simulink model "Sample594"  (R2021b)
settings: Solver=VariableStepAuto  StartTime=0.0  StopTime=10.0  RelTol=1e-3
undefined symbols (not defined in the file): DiscIntNeverNeededParam, magnitude, Newton, Raphson
libraries: simulink x402, pid_lib x98
(part 4 of 14)

== system Sample594/cfblk7/cfblk12/cfblk8 ==
  cfblk1 : Inport
  cfblk8 : Inport  Port=2
  cfblk10 : Subsystem  TreatAsAtomicUnit=on
  cfblk{11..14} (4 alike) : Delay  SampleTime=1
  cfblk3 : simulink/Discrete/Transfer Fcn Lead or Lag  PoleZ=0.95  ZeroZ=0.75  ICPrevOutput=0.0  ICPrevInput=0.0  DoSatur=off
      settings: SourceProductBaseCode=SL
  cfblk4 : DiscreteFir  SampleTime=1
  cfblk5 : Bias  Bias=[232401937.403829]
  cfblk6 : Subsystem
  cfblk7 : If  IfExpression=u1 >= 0  SampleTime=1
  cfblk9 : Subsystem  TreatAsAtomicUnit=on
  cfblk2 : Outport
  wires:
  cfblk1/1 -> cfblk5/1
  cfblk8/1 -> cfblk3/1
  cfblk5/1 -> cfblk4/1, cfblk9/3(cfblk7)
  cfblk3/1 -> cfblk2/1
  cfblk9/1(cfblk2) -> cfblk6/1(cfblk1)
  cfblk4/1 -> cfblk9/2(cfblk6)
  cfblk6/1(cfblk2) -> cfblk11/1, cfblk14/1
  cfblk7/1 -> cfblk9/Action
  cfblk7/2 -> cfblk10/Action
  cfblk11/1 -> cfblk10/1(cfblk1)
  cfblk10/1(cfblk2) -> cfblk12/1
  cfblk12/1 -> cfblk9/1(cfblk1)
  cfblk10/2(cfblk10) -> cfblk13/1
  cfblk13/1 -> cfblk7/1
  cfblk14/1 -> cfblk9/4(cfblk8)

== system Sample594/cfblk7/cfblk12/cfblk9 ==
  cfblk1 : Inport
  cfblk10 : Inport  Port=2
  cfblk11 : Delay  SampleTime=1
  cfblk12 : Delay  SampleTime=1
  cfblk3 : simulink/Discrete/Transfer Fcn First Order  PoleZ=0.95  ICPrevOutput=0.0  DoSatur=off
  cfblk4 : simulink/Discrete/Transfer Fcn First Order  PoleZ=0.95  ICPrevOutput=0.0  DoSatur=off
  cfblk5 : Gain  Gain=[219422416.424969]
  cfblk6 : Polyval  Coefs=[ +2.081618890e-019, -1.441693666e-014, +4.719686976e-010, -8.536869453e-006, +1.621573104e-001, -8.087801117e+001 ]
  cfblk7 : Rounding
  cfblk8 : Constant  Value=[284617864.400396]  SampleTime=1
  cfblk9 : Subsystem
  cfblk2 : Outport
  wires:
  cfblk3/1 -> cfblk5/1
  cfblk1/1 -> cfblk3/1
  cfblk9/1(cfblk2) -> cfblk7/1
  cfblk4/1 -> cfblk9/1(cfblk1)
  cfblk7/1 -> cfblk6/1
  cfblk8/1 -> cfblk2/1
  cfblk6/1 -> cfblk11/1
  cfblk11/1 -> cfblk9/2(cfblk12)
  cfblk9/2(cfblk13) -> cfblk12/1
  cfblk12/1 -> cfblk4/1

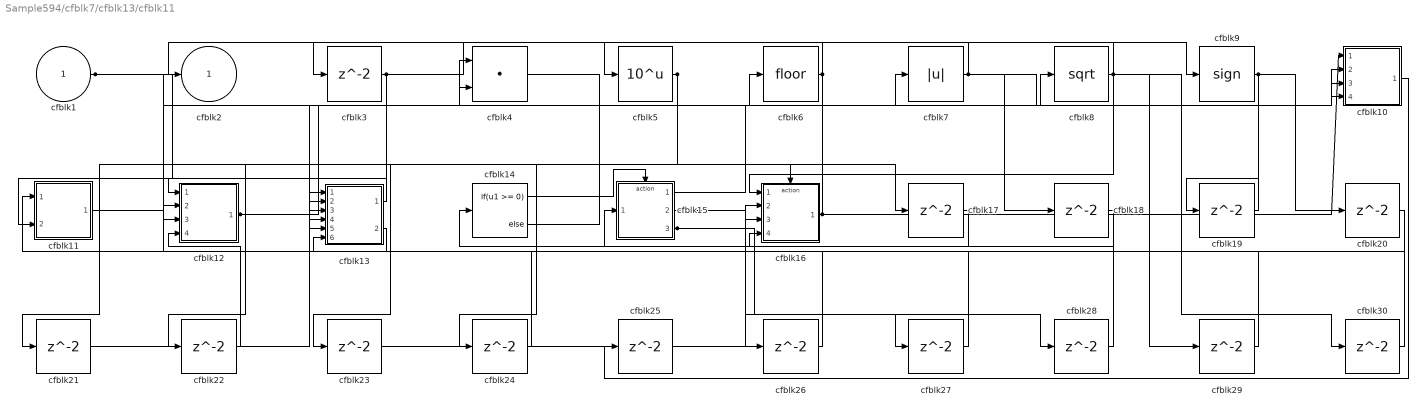
== system Sample594/cfblk7/cfblk13/cfblk11 ==
  cfblk1 : Inport
  cfblk10 : Subsystem
  cfblk11 : Subsystem
  cfblk12 : Subsystem
  cfblk13 : Subsystem
  cfblk14 : If  IfExpression=u1 >= 0  SampleTime=1
  cfblk15 : Subsystem  TreatAsAtomicUnit=on
  cfblk16 : Subsystem  TreatAsAtomicUnit=on
  cfblk{3,17..30} (15 alike) : Delay  SampleTime=1
  cfblk4 : DotProduct  InputSameDT=on  OutDataTypeStr=Inherit: Inherit via internal rule
  cfblk5 : Math  Operator=10^u  SaturateOnIntegerOverflow=on
  cfblk6 : Rounding
  cfblk7 : Abs
  cfblk8 : Sqrt  SaturateOnIntegerOverflow=on
  cfblk9 : Signum
  cfblk2 : Outport
  wires:
  cfblk12/1(cfblk2) -> cfblk8/1, cfblk10/2(cfblk13)
  cfblk8/1 -> cfblk16/1(cfblk1), cfblk2/1, cfblk29/1, cfblk30/1
  cfblk3/1 -> cfblk9/1, cfblk11/2(cfblk7)
  cfblk15/1(cfblk2) -> cfblk7/1
  cfblk16/1(cfblk2) -> cfblk4/1, cfblk10/1(cfblk1)
  cfblk13/1(cfblk2) -> cfblk12/1(cfblk1)
  cfblk13/2(cfblk17) -> cfblk11/1(cfblk1)
  cfblk11/1(cfblk2) -> cfblk6/1
  cfblk6/1 -> cfblk5/1, cfblk21/1, cfblk22/1
  cfblk15/3(cfblk7) -> cfblk27/1, cfblk28/1
  cfblk7/1 -> cfblk3/1, cfblk10/3(cfblk14), cfblk18/1
  cfblk5/1 -> cfblk23/1, cfblk24/1
  cfblk1/1 -> cfblk13/3(cfblk13), cfblk10/4(cfblk15)
  cfblk9/1 -> cfblk19/1, cfblk20/1
  cfblk14/1 -> cfblk15/Action
  cfblk14/2 -> cfblk16/Action
  cfblk4/1 -> cfblk17/1
  cfblk17/1 -> cfblk15/1(cfblk1)
  cfblk18/1 -> cfblk14/1
  cfblk19/1 -> cfblk4/2
  cfblk20/1 -> cfblk13/6(cfblk16)
  cfblk21/1 -> cfblk13/2(cfblk12)
  cfblk22/1 -> cfblk12/4(cfblk14)
  cfblk23/1 -> cfblk16/3(cfblk11)
  cfblk24/1 -> cfblk13/5(cfblk15)
  cfblk10/1(cfblk2) -> cfblk25/1
  cfblk25/1 -> cfblk16/2(cfblk10)
  cfblk15/2(cfblk6) -> cfblk26/1
  cfblk26/1 -> cfblk13/1(cfblk1)
  cfblk27/1 -> cfblk12/2(cfblk12)
  cfblk28/1 -> cfblk16/4(cfblk12)
  cfblk29/1 -> cfblk12/3(cfblk13)
  cfblk30/1 -> cfblk13/4(cfblk14)

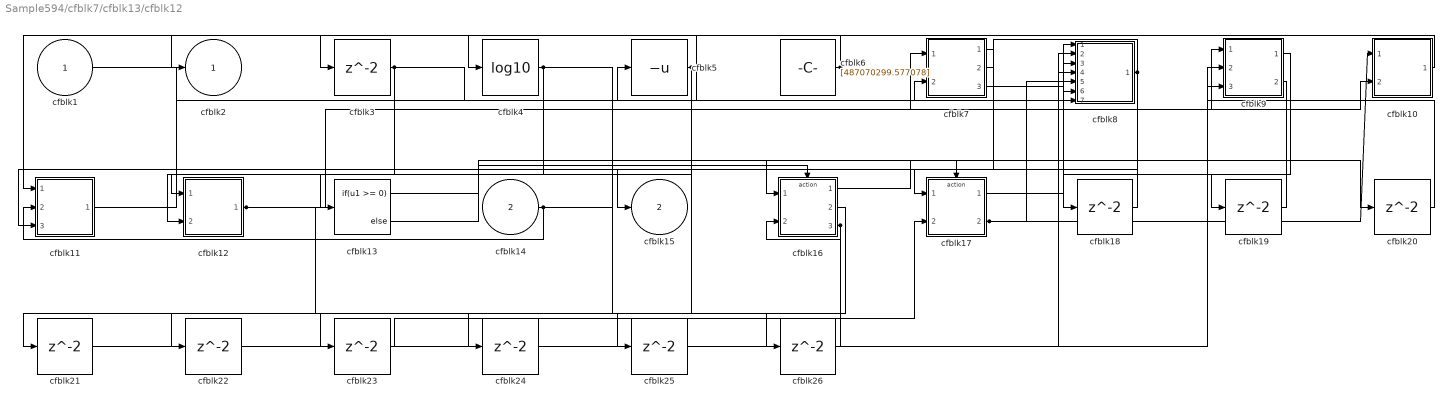
== system Sample594/cfblk7/cfblk13/cfblk12 ==
  cfblk1 : Inport
  cfblk14 : Inport  Port=2
  cfblk10 : Subsystem
  cfblk11 : Subsystem
  cfblk12 : Subsystem
  cfblk13 : If  IfExpression=u1 >= 0  SampleTime=1
  cfblk16 : Subsystem  TreatAsAtomicUnit=on
  cfblk17 : Subsystem  TreatAsAtomicUnit=on
  cfblk{3,18..26} (10 alike) : Delay  SampleTime=1
  cfblk4 : Math  Operator=log10  SaturateOnIntegerOverflow=on
  cfblk5 : UnaryMinus
  cfblk6 : Constant  Value=[487070299.577078]  SampleTime=1
  cfblk7 : Subsystem
  cfblk8 : Subsystem
  cfblk9 : Subsystem
  cfblk2 : Outport
  cfblk15 : Outport  Port=2
  wires:
  cfblk11/1(cfblk2) -> cfblk5/1
  cfblk12/1(cfblk2) -> cfblk9/1(cfblk1), cfblk24/1
  cfblk8/1(cfblk2) -> cfblk11/1(cfblk1), cfblk11/3(cfblk11)
  cfblk17/1(cfblk2) -> cfblk8/1(cfblk1)
  cfblk3/1 -> cfblk13/1, cfblk8/6(cfblk14)
  cfblk1/1 -> cfblk7/2(cfblk9)
  cfblk10/1(cfblk2) -> cfblk4/1
  cfblk6/1 -> cfblk2/1, cfblk3/1
  cfblk16/3(cfblk16) -> cfblk22/1, cfblk23/1
  cfblk4/1 -> cfblk12/1(cfblk1), cfblk26/1
  cfblk5/1 -> cfblk12/2(cfblk7), cfblk25/1
  cfblk7/1(cfblk2) -> cfblk17/1(cfblk1)
  cfblk17/2(cfblk9) -> cfblk10/1(cfblk1), cfblk8/5(cfblk13)
  cfblk14/1 -> cfblk11/2(cfblk10), cfblk10/2(cfblk8)
  cfblk7/2(cfblk10) -> cfblk15/1
  cfblk7/3(cfblk11) -> cfblk8/3(cfblk11)
  cfblk13/1 -> cfblk16/Action
  cfblk13/2 -> cfblk17/Action
  cfblk9/1(cfblk2) -> cfblk18/1
  cfblk18/1 -> cfblk7/1(cfblk1)
  cfblk9/2(cfblk8) -> cfblk19/1
  cfblk19/1 -> cfblk16/1(cfblk1)
  cfblk16/1(cfblk2) -> cfblk20/1
  cfblk20/1 -> cfblk9/2(cfblk6)
  cfblk16/2(cfblk15) -> cfblk21/1
  cfblk21/1 -> cfblk9/3(cfblk7)
  cfblk22/1 -> cfblk8/2(cfblk10)
  cfblk23/1 -> cfblk17/2(cfblk8)
  cfblk24/1 -> cfblk8/7(cfblk15)
  cfblk25/1 -> cfblk8/4(cfblk12)
  cfblk26/1 -> cfblk16/2(cfblk14)

== system Sample594/cfblk7/cfblk13/cfblk17 ==
  cfblk1 : Inport
  Action Port : ActionPort  ActionPortLabel=if(u1 >= 0)
  cfblk10 : Subsystem
  cfblk11 : Subsystem
  cfblk12 : Subsystem
  cfblk13 : Subsystem
  cfblk15 : Delay
  cfblk16 : Delay
  cfblk17 : Delay
  cfblk3 : simulink/Discrete/Difference  ICPrevInput=0.0  OutMin=[]  OutMax=[]  OutDataTypeStr=Inherit: Inherit via back propagation  OutDataType=fixdt(1, 16)  OutScaling=2^-10  DoSatur=off
  cfblk4 : DiscreteTransferFcn
  cfblk5 : Reshape
  cfblk6 : simulink/Math Operations/Slider Gain  gain=1  low=0  high=2
  cfblk7 : DotProduct  InputSameDT=on  OutDataTypeStr=Inherit: Inherit via internal rule
  cfblk8 : Constant  Value=[310623050.660394]  SampleTime=1
  cfblk9 : Subsystem
  cfblk2 : Outport
  cfblk14 : Outport  Port=2
  wires:
  cfblk6/1 -> cfblk11/1(cfblk1)
  cfblk13/1(cfblk2) -> cfblk3/1
  cfblk7/1 -> cfblk15/1, cfblk16/1
  cfblk3/1 -> cfblk2/1, cfblk7/2
  cfblk12/1(cfblk2) -> cfblk4/1, cfblk13/3(cfblk7)
  cfblk10/1(cfblk2) -> cfblk11/2(cfblk12)
  cfblk1/1 -> cfblk5/1, cfblk6/1, cfblk12/3(cfblk16)
  cfblk4/1 -> cfblk13/1(cfblk1), cfblk9/1(cfblk1)
  cfblk9/1(cfblk2) -> cfblk14/1
  cfblk11/1(cfblk2) -> cfblk12/1(cfblk1)
  cfblk5/1 -> cfblk10/2(cfblk7)
  cfblk8/1 -> cfblk13/2(cfblk6)
  cfblk9/3(cfblk10) -> cfblk7/1
  cfblk15/1 -> cfblk10/1(cfblk1)
  cfblk16/1 -> cfblk12/2(cfblk15)
  cfblk9/2(cfblk9) -> cfblk17/1
  cfblk17/1 -> cfblk11/3(cfblk13)

== system Sample594/cfblk7/cfblk13/cfblk18 ==
  cfblk1 : Inport
  Action Port : ActionPort  ActionPortLabel=else
  cfblk{9..12} (4 alike) : Delay
  cfblk3 : pid_lib/PID Controller  Controller=PID  Form=Parallel  TimeDomain=Discrete-time  UseExternalTs=off  SampleTime=-1  IntegratorMethod=Forward Euler  FilterMethod=Forward Euler  ControllerParametersSource=internal  P=1  I=1  D=0  UseFilter=on  N=100  TunerSelectOption=Transfer Function Based (PID Tuner App)  InitialConditionSource=internal  InitialConditionForIntegrator=0  InitialConditionForFilter=0  DifferentiatorICPrevScaledInput=0  ExternalReset=none  TrackingMode=off  Kt=1  LimitOutput=off  SatLimitsSource=internal  UpperSaturationLimit=inf  LowerSaturationLimit=-inf  LinearizeAsGain=off  AntiWindupMode=none  Kb=1  POutMin=[]  POutMax=[]  IOutMin=[]  IOutMax=[]  DOutMin=[]  DOutMax=[]  NOutMin=[]  NOutMax=[]  SumOutMin=[]  SumOutMax=[]  SaturationOutMin=[]  SaturationOutMax=[]  PParamMin=[]  PParamMax=[]  IParamMin=[]  IParamMax=[]  DParamMin=[]  DParamMax=[]  NParamMin=[]  NParamMax=[]  KbParamMin=[]  KbParamMax=[]  KtParamMin=[]  KtParamMax=[]  KbOutMin=[]  KbOutMax=[]  KtOutMin=[]  KtOutMax=[]  IntegratorOutMin=[]  IntegratorOutMax=[]  FilterOutMin=[]  FilterOutMax=[]  SumI1OutMin=[]  SumI1OutMax=[]  SumI2OutMin=[]  SumI2OutMax=[]  SumI3OutMin=[]  SumI3OutMax=[]  SumI4OutMin=[]  SumI4OutMax=[]  SumDOutMin=[]  SumDOutMax=[]  DifferentiatorOutMin=[]  DifferentiatorOutMax=[]  FilterDiffOutCoefMin=[]  FilterDiffOutCoefMax=[]  ReciprocalOutMin=[]  ReciprocalOutMax=[]  SumDenOutMin=[]  SumDenOutMax=[]  SumNumOutMin=[]  SumNumOutMax=[]  DivideOutMin=[]  DivideOutMax=[]  UdiffTsProdOutMin=[]  UdiffTsProdOutMax=[]  NTsProdOutMin=[]  NTsProdOutMax=[]  UintegralTsProdOutMin=[]  UintegralTsProdOutMax=[]  UngainTsProdOutMin=[]  UngainTsProdOutMax=[]  IntegratorContinuousStateAttributes=''  IntegratorStateMustResolveToSignalObject=off  IntegratorRTWStateStorageClass=Auto  FilterContinuousStateAttributes=''  FilterStateMustResolveToSignalObject=off  FilterRTWStateStorageClass=Auto  ParallelPVariant=InternalParameters  IdealPVariant=Disabled  IVariant=InternalParameters  DVariant=InternalParameters  IntegratorVariant=Discrete  SatVariant=Disabled  AWVariant=Passthrough  PCopyVariant=Disabled  TRVariant=Disabled  FdbkBlocksVariant=Forward  IdealPFdbkVariant=Disabled  SatFdbkVariant=Disabled  DerivativeFilterVariant=ForwardEulerFilter  NVariant=InternalParameters  NCopyVariant=Disabled  FilterICVariant=InternalICsFilter  IntegratorICVariant=InternalICs  ExternalResetVariant=Disabled  TRSumVariant=Passthrough  SumFdbkVariant=Disabled  SumVariant=Sum_PID  TsampFilterVariant=InternalTs  TsampNgainVariant=Passthrough  TsampIntegralVariant=Passthrough  ExternalSaturationOutDataTypeStr=Inherit: Same as second input
  cfblk4 : Assignment  DiagnosticForDimensions=Warning  IndexOptions=Index vector (dialog)  Indices=1  OutputSizes=1
  cfblk5 : Subsystem
  cfblk6 : Subsystem
  cfblk7 : Subsystem
  cfblk8 : Subsystem
  cfblk2 : Outport
  wires:
  cfblk1/1 -> cfblk5/1(cfblk1)
  cfblk7/1(cfblk2) -> cfblk4/2, cfblk9/1
  cfblk8/1(cfblk2) -> cfblk7/1(cfblk1), cfblk6/3(cfblk6)
  cfblk5/1(cfblk2) -> cfblk8/2(cfblk9)
  cfblk5/2(cfblk11) -> cfblk6/1(cfblk1), cfblk6/2(cfblk5), cfblk7/2(cfblk7), cfblk7/3(cfblk8), cfblk7/4(cfblk9)
  cfblk6/2(cfblk7) -> cfblk2/1, cfblk3/1, cfblk4/1
  cfblk9/1 -> cfblk5/3(cfblk9)
  cfblk4/1 -> cfblk10/1
  cfblk10/1 -> cfblk5/2(cfblk8)
  cfblk6/1(cfblk2) -> cfblk11/1
  cfblk11/1 -> cfblk8/1(cfblk1)
  cfblk3/1 -> cfblk12/1
  cfblk12/1 -> cfblk5/4(cfblk10)

== system Sample594/cfblk7/cfblk17/cfblk8 ==
  cfblk1 : Inport
  cfblk10 : MinMax  Function=max  Inputs=3
  cfblk11 : Gain  Gain=[-356507921.559494]
  cfblk12 : Constant  Value=[-799910356.310316]  SampleTime=1
  cfblk13 : Subsystem
  cfblk14 : Subsystem
  cfblk{15..18} (4 alike) : Delay
  cfblk3 : UnitDelay  SampleTime=-1  HasFrameUpgradeWarning=on
  cfblk4 : DiscreteStateSpace  SampleTime=-1
  cfblk5 : UnitDelay  SampleTime=-1  HasFrameUpgradeWarning=on
  cfblk6 : DiscreteStateSpace  SampleTime=-1
  cfblk7 : simulink/Discrete/Difference  ICPrevInput=0.0  OutMin=[]  OutMax=[]  OutDataTypeStr=Inherit: Inherit via back propagation  OutDataType=fixdt(1, 16)  OutScaling=2^-10  DoSatur=off
  cfblk8 : Gain  Gain=[-919229611.126287]
  cfblk9 : ComplexToMagnitudeAngle
  cfblk2 : Outport
  wires:
  cfblk5/1 -> cfblk6/1
  cfblk12/1 -> cfblk10/1
  cfblk4/1 -> cfblk7/1, cfblk11/1
  cfblk9/1 -> cfblk4/1
  cfblk3/1 -> cfblk14/1(cfblk1), cfblk13/3(cfblk14)
  cfblk11/1 -> cfblk10/2
  cfblk7/1 -> cfblk5/1
  cfblk8/1 -> cfblk13/2(cfblk13), cfblk18/1
  cfblk13/1(cfblk2) -> cfblk10/3
  cfblk9/2 -> cfblk8/1
  cfblk14/1(cfblk2) -> cfblk9/1
  cfblk6/1 -> cfblk13/1(cfblk1)
  cfblk1/1 -> cfblk2/1
  cfblk10/1 -> cfblk15/1
  cfblk15/1 -> cfblk3/1
  cfblk13/2(cfblk15) -> cfblk16/1
  cfblk16/1 -> cfblk14/3(cfblk10)
  cfblk13/3(cfblk16) -> cfblk17/1
  cfblk17/1 -> cfblk14/4(cfblk11)
  cfblk18/1 -> cfblk14/2(cfblk9)

== system Sample594/cfblk7/cfblk18/cfblk10 ==
  cfblk1 : Inport
  cfblk14 : Inport  Port=2
  cfblk15 : Inport  Port=3
  cfblk10 : Product
  cfblk11 : ComplexToMagnitudeAngle
  cfblk12 : Sqrt  Operator=rSqrt  AlgorithmType=Newton-Raphson  SaturateOnIntegerOverflow=on
  cfblk13 : Subsystem
  cfblk16 : Delay
  cfblk17 : Delay
  cfblk18 : Delay
  cfblk3 : Delay  ShowEnablePort=on
      settings: InputPortMap=u0,e6
  cfblk4 : simulink/Discrete/Transfer Fcn First Order  PoleZ=0.95  ICPrevOutput=0.0  DoSatur=off
  cfblk5 : DiscreteStateSpace  SampleTime=-1
  cfblk6 : DiscreteZeroPole  Poles=[0 0.5]  Gain=1  SampleTime=-1
  cfblk7 : DiscreteTransferFcn
  cfblk8 : Assignment  DiagnosticForDimensions=Warning  IndexOptions=Index vector (dialog)  Indices=1  OutputSizes=1
  cfblk9 : Sum  Inputs=+
  cfblk2 : Outport
  wires:
  cfblk13/1(cfblk2) -> cfblk5/1
  cfblk7/1 -> cfblk8/1
  cfblk6/1 -> cfblk9/1
  cfblk3/1 -> cfblk11/1
  cfblk10/1 -> cfblk6/1
  cfblk9/1 -> cfblk12/1
  cfblk5/1 -> cfblk7/1
  cfblk12/1 -> cfblk13/1(cfblk1)
  cfblk11/2 -> cfblk4/1
  cfblk8/1 -> cfblk3/2, cfblk17/1
  cfblk15/1 -> cfblk13/2(cfblk6)
  cfblk14/1 -> cfblk8/2
  cfblk4/1 -> cfblk2/1
  cfblk1/1 -> cfblk10/1
  cfblk11/1 -> cfblk16/1
  cfblk16/1 -> cfblk3/1
  cfblk17/1 -> cfblk13/3(cfblk7)
  cfblk13/2(cfblk8) -> cfblk18/1
  cfblk18/1 -> cfblk10/2

== system Sample594/cfblk7/cfblk18/cfblk9 ==
  cfblk1 : Inport
  cfblk10 : Subsystem
  cfblk3 : Delay  ShowEnablePort=on
      settings: InputPortMap=u0,e6
  cfblk4 : ComplexToRealImag
  cfblk5 : Abs
  cfblk6 : ComplexToMagnitudeAngle
  cfblk7 : Constant  Value=[389657295.438685]  SampleTime=1
  cfblk8 : Constant  Value=[-589872672.868971]  SampleTime=1
  cfblk9 : Constant  Value=[-970659271.621519]  SampleTime=1
  cfblk2 : Outport
  wires:
  cfblk4/1 -> cfblk3/1
  cfblk7/1 -> cfblk2/1
  cfblk8/1 -> cfblk5/1
  cfblk9/1 -> cfblk3/2
  cfblk5/1 -> cfblk10/1(cfblk1)
  cfblk1/1 -> cfblk6/1
  cfblk10/1(cfblk2) -> cfblk4/1

== system Sample594/cfblk7/cfblk19/cfblk7 ==
  cfblk1 : Inport
  cfblk11 : Inport  Port=2
  cfblk12 : Inport  Port=3
  cfblk10 : Constant  Value=[-662759039.871267]  SampleTime=1
  cfblk3 : simulink/Discrete/Transfer Fcn Real Zero  ZeroZ=0.75  ICPrevInput=0.0  DoSatur=off
      settings: SourceProductBaseCode=SL
  cfblk4 : simulink/Discrete/Difference  ICPrevInput=0.0  OutMin=[]  OutMax=[]  OutDataTypeStr=Inherit: Inherit via back propagation  OutDataType=fixdt(1, 16)  OutScaling=2^-10  DoSatur=off
  cfblk5 : Product  Inputs=**
  cfblk6 : ComplexToMagnitudeAngle
  cfblk7 : Sum  Inputs=|++
  cfblk8 : MinMax  Function=max  Inputs=3
  cfblk9 : Sum
  cfblk2 : Outport
  cfblk13 : Outport  Port=2
  cfblk14 : Outport  Port=3
  cfblk15 : Outport  Port=4
  wires:
  cfblk4/1 -> cfblk8/1
  cfblk11/1 -> cfblk7/1, cfblk9/2
  cfblk5/1 -> cfblk15/1
  cfblk9/1 -> cfblk7/2
  cfblk8/1 -> cfblk2/1
  cfblk12/1 -> cfblk8/2
  cfblk1/1 -> cfblk3/1
  cfblk10/1 -> cfblk9/1, cfblk8/3
  cfblk3/1 -> cfblk13/1, cfblk14/1
  cfblk7/1 -> cfblk6/1, cfblk4/1
  cfblk6/1 -> cfblk5/1
  cfblk6/2 -> cfblk5/2

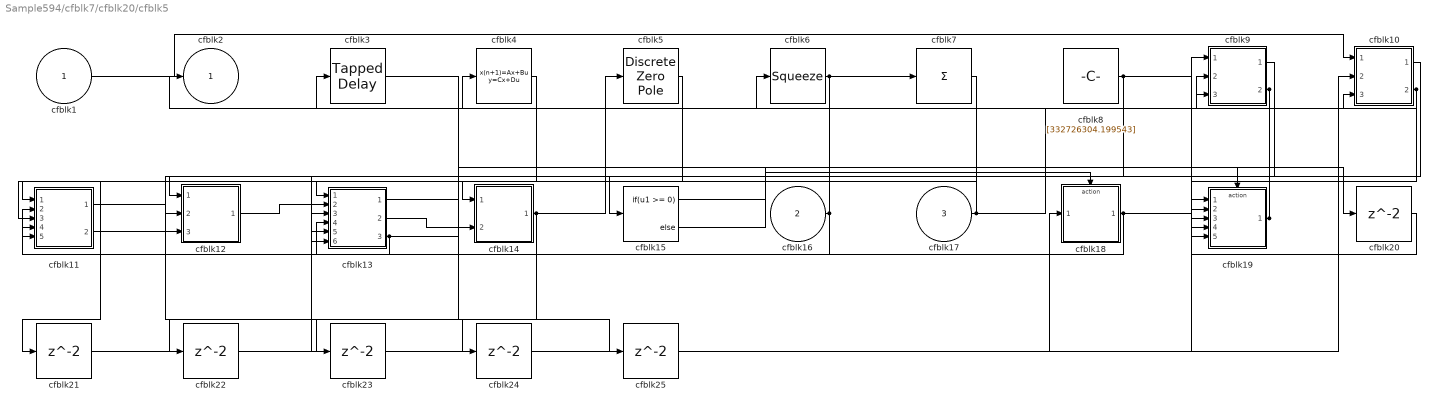
== system Sample594/cfblk7/cfblk20/cfblk5 ==
  cfblk1 : Inport
  cfblk16 : Inport  Port=2
  cfblk17 : Inport  Port=3
  cfblk10 : Subsystem
  cfblk11 : Subsystem
  cfblk12 : Subsystem
  cfblk13 : Subsystem
  cfblk14 : Subsystem
  cfblk15 : If  IfExpression=u1 >= 0  SampleTime=1
  cfblk18 : Subsystem  TreatAsAtomicUnit=on
  cfblk19 : Subsystem  TreatAsAtomicUnit=on
  cfblk{20..25} (6 alike) : Delay
  cfblk3 : simulink/Discrete/Tapped Delay  vinit=0.0  samptime=-1  NumDelays=1  DelayOrder=Oldest  includeCurrent=off
  cfblk4 : DiscreteStateSpace  SampleTime=-1
  cfblk5 : DiscreteZeroPole  Poles=[0 0.5]  Gain=1  SampleTime=-1
  cfblk6 : Squeeze
  cfblk7 : Sum  Inputs=+
  cfblk8 : Constant  Value=[332726304.199543]  SampleTime=1
  cfblk9 : Subsystem
  cfblk2 : Outport
  wires:
  cfblk10/1(cfblk2) -> cfblk15/1
  cfblk8/1 -> cfblk19/2(cfblk8), cfblk12/3(cfblk17)
  cfblk14/1(cfblk2) -> cfblk5/1, cfblk22/1
  cfblk16/1 -> cfblk13/1(cfblk1), cfblk12/2(cfblk16), cfblk11/4(cfblk13)
  cfblk6/1 -> cfblk7/1, cfblk11/1(cfblk1), cfblk11/3(cfblk12)
  cfblk1/1 -> cfblk10/1(cfblk1)
  cfblk19/1(cfblk2) -> cfblk9/2(cfblk12), cfblk4/1
  cfblk12/1(cfblk2) -> cfblk13/2(cfblk10)
  cfblk17/1 -> cfblk2/1, cfblk10/3(cfblk16)
  cfblk7/1 -> cfblk14/1(cfblk1)
  cfblk9/1(cfblk2) -> cfblk12/1(cfblk1)
  cfblk13/2(cfblk15) -> cfblk14/2(cfblk10)
  cfblk4/1 -> cfblk13/3(cfblk11)
  cfblk13/3(cfblk16) -> cfblk6/1, cfblk11/2(cfblk11), cfblk11/5(cfblk14)
  cfblk18/1(cfblk2) -> cfblk19/4(cfblk10), cfblk13/4(cfblk12)
  cfblk10/2(cfblk17) -> cfblk9/3(cfblk13), cfblk19/5(cfblk11)
  cfblk9/2(cfblk14) -> cfblk3/1, cfblk13/6(cfblk14)
  cfblk15/1 -> cfblk18/Action
  cfblk15/2 -> cfblk19/Action
  cfblk13/1(cfblk2) -> cfblk20/1
  cfblk20/1 -> cfblk19/3(cfblk9)
  cfblk5/1 -> cfblk21/1
  cfblk21/1 -> cfblk10/2(cfblk15)
  cfblk22/1 -> cfblk13/5(cfblk13)
  cfblk11/1(cfblk2) -> cfblk23/1
  cfblk23/1 -> cfblk19/1(cfblk1)
  cfblk11/2(cfblk15) -> cfblk24/1
  cfblk24/1 -> cfblk18/1(cfblk1)
  cfblk3/1 -> cfblk25/1
  cfblk25/1 -> cfblk9/1(cfblk1)

== system Sample594/cfblk7/cfblk20/cfblk6 ==
  cfblk1 : Inport
  cfblk6 : Inport  Port=2
  cfblk7 : Inport  Port=3
  cfblk8 : Inport  Port=4
  cfblk9 : Inport  Port=5
  cfblk3 : DiscreteFilter
  cfblk4 : Delay
  cfblk5 : Constant  Value=[-339919345.684127]  SampleTime=1
  cfblk2 : Outport
  cfblk10 : Outport  Port=2
  wires:
  cfblk9/1 -> cfblk10/1
  cfblk3/1 -> cfblk2/1
  cfblk1/1 -> cfblk3/1
  cfblk5/1 -> cfblk4/1

== system Sample594/cfblk7/cfblk8/cfblk10 ==
  cfblk1 : Inport
  cfblk10 : Inport  Port=2
  cfblk{12..15} (4 alike) : Delay  SampleTime=1
  cfblk3 : DiscreteStateSpace
  cfblk4 : Reshape
  cfblk5 : Sum  Inputs=+
  cfblk6 : Signum
  cfblk7 : Subsystem
  cfblk8 : Subsystem
  cfblk9 : Subsystem
  cfblk2 : Outport
  cfblk11 : Outport  Port=2
  wires:
  cfblk1/1 -> cfblk11/1
  cfblk9/1(cfblk2) -> cfblk4/1
  cfblk5/1 -> cfblk6/1, cfblk13/1
  cfblk9/2(cfblk15) -> cfblk2/1
  cfblk3/1 -> cfblk9/1(cfblk1)
  cfblk7/1(cfblk2) -> cfblk8/1(cfblk1)
  cfblk4/1 -> cfblk7/2(cfblk9), cfblk15/1
  cfblk10/1 -> cfblk9/3(cfblk13)
  cfblk8/2(cfblk7) -> cfblk5/1
  cfblk9/3(cfblk16) -> cfblk8/2(cfblk6)
  cfblk8/1(cfblk2) -> cfblk12/1
  cfblk12/1 -> cfblk9/2(cfblk12)
  cfblk13/1 -> cfblk3/1
  cfblk6/1 -> cfblk14/1
  cfblk14/1 -> cfblk7/1(cfblk1)
  cfblk15/1 -> cfblk9/4(cfblk14)

== system Sample594/cfblk7/cfblk8/cfblk11 ==
  cfblk1 : Inport
  cfblk{10..14} (5 alike) : Delay  SampleTime=1
  cfblk3 : DiscreteZeroPole  Poles=[0 0.5]  Gain=1
  cfblk4 : simulink/Discrete/Tapped Delay  vinit=0.0  samptime=-1  NumDelays=1  DelayOrder=Oldest  includeCurrent=off
  cfblk5 : PermuteDimensions
  cfblk6 : Abs
  cfblk7 : Product  Inputs=*
  cfblk8 : Subsystem
  cfblk9 : Subsystem
  cfblk2 : Outport
  wires:
  cfblk4/1 -> cfblk9/1(cfblk1)
  cfblk1/1 -> cfblk2/1
  cfblk9/1(cfblk2) -> cfblk6/1
  cfblk7/1 -> cfblk4/1, cfblk11/1, cfblk12/1, cfblk13/1
  cfblk8/1(cfblk2) -> cfblk5/1
  cfblk3/1 -> cfblk8/1(cfblk1), cfblk9/4(cfblk13)
  cfblk5/1 -> cfblk7/1, cfblk14/1
  cfblk8/2(cfblk16) -> cfblk9/2(cfblk11)
  cfblk8/3(cfblk17) -> cfblk9/3(cfblk12)
  cfblk6/1 -> cfblk10/1
  cfblk10/1 -> cfblk3/1
  cfblk11/1 -> cfblk8/2(cfblk12)
  cfblk12/1 -> cfblk8/3(cfblk13)
  cfblk13/1 -> cfblk8/4(cfblk14)
  cfblk14/1 -> cfblk8/5(cfblk15)

== system Sample594/cfblk7/cfblk8/cfblk12 ==
  cfblk1 : Inport
  cfblk17 : Inport  Port=2
  cfblk10 : Sum  Inputs=+-
  cfblk11 : Abs
  cfblk12 : Constant  Value=[25573350.460328]  SampleTime=1
  cfblk13 : Subsystem
  cfblk14 : Subsystem
  cfblk15 : Subsystem
  cfblk16 : Subsystem
  cfblk18 : Delay  SampleTime=1
  cfblk19 : Delay  SampleTime=1
  cfblk20 : Delay  SampleTime=1
  cfblk3 : simulink/Discrete/Transfer Fcn Lead or Lag  PoleZ=0.95  ZeroZ=0.75  ICPrevOutput=0.0  ICPrevInput=0.0  DoSatur=off
      settings: SourceProductBaseCode=SL
  cfblk4 : UnitDelay  HasFrameUpgradeWarning=on
  cfblk5 : DiscreteFir  SampleTime=1
  cfblk6 : Sum  Inputs=+
  cfblk7 : Assignment  DiagnosticForDimensions=Warning  IndexOptions=Index vector (dialog)  Indices=1  OutputSizes=1
  cfblk8 : Sqrt  SaturateOnIntegerOverflow=on
  cfblk9 : ComplexToMagnitudeAngle
  cfblk2 : Outport
  wires:
  cfblk9/1 -> cfblk2/1
  cfblk5/1 -> cfblk11/1
  cfblk6/1 -> cfblk16/1(cfblk1)
  cfblk13/1(cfblk2) -> cfblk6/1
  cfblk10/1 -> cfblk9/1
  cfblk8/1 -> cfblk10/1
  cfblk12/1 -> cfblk14/1(cfblk1)
  cfblk3/1 -> cfblk8/1
  cfblk14/1(cfblk2) -> cfblk13/1(cfblk1)
  cfblk1/1 -> cfblk10/2
  cfblk14/2(cfblk9) -> cfblk15/1(cfblk1)
  cfblk15/1(cfblk2) -> cfblk7/1
  cfblk7/1 -> cfblk5/1
  cfblk9/2 -> cfblk7/2
  cfblk4/1 -> cfblk14/3(cfblk6)
  cfblk16/1(cfblk2) -> cfblk3/1
  cfblk17/1 -> cfblk14/4(cfblk7)
  cfblk13/2(cfblk12) -> cfblk18/1
  cfblk18/1 -> cfblk14/2(cfblk5)
  cfblk15/2(cfblk6) -> cfblk19/1
  cfblk19/1 -> cfblk4/1
  cfblk15/3(cfblk7) -> cfblk20/1
  cfblk20/1 -> cfblk14/5(cfblk8)

== system Sample594/cfblk7/cfblk8/cfblk13 ==
  cfblk1 : Inport
  cfblk{10..13} (4 alike) : Delay  SampleTime=1
  cfblk3 : Trigonometry
  cfblk4 : Polyval  Coefs=[ +2.081618890e-019, -1.441693666e-014, +4.719686976e-010, -8.536869453e-006, +1.621573104e-001, -8.087801117e+001 ]
  cfblk5 : simulink/Math Operations/MinMax Running Resettable  Function=min  vinit=0.0
  cfblk6 : Subsystem
  cfblk7 : Subsystem
  cfblk8 : Subsystem
  cfblk9 : Subsystem
  cfblk2 : Outport
  wires:
  cfblk5/1 -> cfblk8/1(cfblk1)
  cfblk9/1(cfblk2) -> cfblk6/1(cfblk1)
  cfblk4/1 -> cfblk2/1
  cfblk3/1 -> cfblk7/3(cfblk16), cfblk11/1
  cfblk1/1 -> cfblk5/2, cfblk8/3(cfblk15)
  cfblk6/1(cfblk2) -> cfblk4/1
  cfblk8/1(cfblk2) -> cfblk9/1(cfblk1), cfblk9/3(cfblk8), cfblk7/4(cfblk17)
  cfblk9/2(cfblk9) -> cfblk6/3(cfblk15)
  cfblk6/2(cfblk16) -> cfblk3/1, cfblk7/1(cfblk1), cfblk7/2(cfblk15), cfblk10/1
  cfblk10/1 -> cfblk9/2(cfblk7)
  cfblk11/1 -> cfblk5/1
  cfblk7/1(cfblk2) -> cfblk12/1
  cfblk12/1 -> cfblk6/2(cfblk14)
  cfblk9/3(cfblk10) -> cfblk13/1
  cfblk13/1 -> cfblk8/2(cfblk14)

== system Sample594/cfblk7/cfblk8/cfblk14 ==
  cfblk1 : Inport
  cfblk6 : Inport  Port=2
  cfblk7 : Inport  Port=3
  cfblk10 : Delay  SampleTime=1
  cfblk11 : Delay  SampleTime=1
  cfblk3 : Bias  Bias=[-355088403.272732]
  cfblk4 : Sin  TimeSource=Use external signal  SampleTime=0
  cfblk5 : Subsystem
  cfblk2 : Outport
  cfblk8 : Outport  Port=2
  cfblk9 : Outport  Port=3
  wires:
  cfblk6/1 -> cfblk3/1
  cfblk4/1 -> cfblk10/1, cfblk11/1
  cfblk3/1 -> cfblk9/1, cfblk5/3(cfblk12)
  cfblk7/1 -> cfblk5/2(cfblk11)
  cfblk1/1 -> cfblk8/1, cfblk5/4(cfblk13)
  cfblk5/1(cfblk2) -> cfblk4/1
  cfblk5/2(cfblk15) -> cfblk2/1
  cfblk10/1 -> cfblk5/1(cfblk1)
  cfblk11/1 -> cfblk5/5(cfblk14)

== system Sample594/cfblk7/cfblk9/cfblk6 ==
  cfblk1 : Inport
  cfblk15 : Inport  Port=2
  cfblk16 : Inport  Port=3
  cfblk17 : Inport  Port=4
  cfblk10 : Product  Inputs=**
  cfblk11 : Constant  Value=[471606698.671259]  SampleTime=1
  cfblk12 : Constant  Value=[-698030242.211273]  SampleTime=1
  cfblk13 : Subsystem
  cfblk14 : Subsystem
  cfblk18 : Delay  SampleTime=1
  cfblk19 : Delay  SampleTime=1
  cfblk3 : Delay  ShowEnablePort=on  SampleTime=1
      settings: InputPortMap=u0,e6
  cfblk4 : pid_lib/PID Controller (2DOF)  Controller=PID  Form=Parallel  TimeDomain=Discrete-time  UseExternalTs=off  SampleTime=1  IntegratorMethod=Forward Euler  FilterMethod=Forward Euler  ControllerParametersSource=internal  P=1  I=1  D=0  UseFilter=on  N=100  b=1  c=1  TunerSelectOption=Transfer Function Based (PID Tuner App)  InitialConditionSource=internal  InitialConditionForIntegrator=0  InitialConditionForFilter=0  DifferentiatorICPrevScaledInput=0  ExternalReset=none  TrackingMode=off  Kt=1  LimitOutput=off  SatLimitsSource=internal  UpperSaturationLimit=inf  LowerSaturationLimit=-inf  LinearizeAsGain=off  AntiWindupMode=none  Kb=1  POutMin=[]  POutMax=[]  IOutMin=[]  IOutMax=[]  DOutMin=[]  DOutMax=[]  NOutMin=[]  NOutMax=[]  bOutMin=[]  bOutMax=[]  cOutMin=[]  cOutMax=[]  SumOutMin=[]  SumOutMax=[]  SaturationOutMin=[]  SaturationOutMax=[]  PParamMin=[]  PParamMax=[]  IParamMin=[]  IParamMax=[]  DParamMin=[]  DParamMax=[]  NParamMin=[]  NParamMax=[]  bParamMin=[]  bParamMax=[]  cParamMin=[]  cParamMax=[]  KbParamMin=[]  KbParamMax=[]  KtParamMin=[]  KtParamMax=[]  KbOutMin=[]  KbOutMax=[]  KtOutMin=[]  KtOutMax=[]  IntegratorOutMin=[]  IntegratorOutMax=[]  FilterOutMin=[]  FilterOutMax=[]  SumI1OutMin=[]  SumI1OutMax=[]  SumI2OutMin=[]  SumI2OutMax=[]  SumI3OutMin=[]  SumI3OutMax=[]  SumI4OutMin=[]  SumI4OutMax=[]  SumDOutMin=[]  SumDOutMax=[]  Sum1OutMin=[]  Sum1OutMax=[]  Sum2OutMin=[]  Sum2OutMax=[]  Sum3OutMin=[]  Sum3OutMax=[]  DifferentiatorOutMin=[]  DifferentiatorOutMax=[]  FilterDiffOutCoefMin=[]  FilterDiffOutCoefMax=[]  ReciprocalOutMin=[]  ReciprocalOutMax=[]  SumDenOutMin=[]  SumDenOutMax=[]  SumNumOutMin=[]  SumNumOutMax=[]  DivideOutMin=[]  DivideOutMax=[]  UdiffTsProdOutMin=[]  UdiffTsProdOutMax=[]  NTsProdOutMin=[]  NTsProdOutMax=[]  UintegralTsProdOutMin=[]  UintegralTsProdOutMax=[]  UngainTsProdOutMin=[]  UngainTsProdOutMax=[]  IntegratorContinuousStateAttributes=''  IntegratorStateMustResolveToSignalObject=off  IntegratorRTWStateStorageClass=Auto  FilterContinuousStateAttributes=''  FilterStateMustResolveToSignalObject=off  FilterRTWStateStorageClass=Auto  ParallelPVariant=InternalParameters  IdealPVariant=Disabled  IVariant=InternalParameters  DVariant=InternalParameters  bVariant=InternalParameters  cVariant=InternalParameters  IntegratorVariant=Discrete  SatVariant=Disabled  AWVariant=Passthrough  PCopyVariant=Disabled  TRVariant=Disabled  FdbkBlocksVariant=Forward  IdealPFdbkVariant=Disabled  SatFdbkVariant=Disabled  DerivativeFilterVariant=ForwardEulerFilter  NVariant=InternalParameters  NCopyVariant=Disabled  FilterICVariant=InternalICsFilter  IntegratorICVariant=InternalICs  ExternalResetVariant=Disabled  TRSumVariant=Passthrough  SumFdbkVariant=Disabled  SumVariant=Sum_PID  TsampFilterVariant=InternalTs  TsampNgainVariant=Passthrough  TsampIntegralVariant=Passthrough  ExternalSaturationOutDataTypeStr=Inherit: Same as second input
      settings: SourceProductBaseCode=SL
  cfblk5 : DiscreteTransferFcn  SampleTime=1
  cfblk6 : Bias  Bias=[998006296.082053]
  cfblk7 : Assignment  DiagnosticForDimensions=Warning  IndexOptions=Index vector (dialog)  Indices=1  OutputSizes=1
  cfblk8 : Squeeze
  cfblk9 : Sum
  cfblk2 : Outport
  wires:
  cfblk10/1 -> cfblk5/1
  cfblk17/1 -> cfblk13/1(cfblk1)
  cfblk15/1 -> cfblk4/1
  cfblk1/1 -> cfblk2/1
  cfblk8/1 -> cfblk13/2(cfblk11)
  cfblk16/1 -> cfblk8/1
  cfblk14/1(cfblk2) -> cfblk7/1, cfblk9/2
  cfblk12/1 -> cfblk6/1
  cfblk3/1 -> cfblk4/2
  cfblk11/1 -> cfblk3/2
  cfblk6/1 -> cfblk7/2
  cfblk13/1(cfblk2) -> cfblk10/1
  cfblk4/1 -> cfblk10/2
  cfblk13/2(cfblk12) -> cfblk9/1
  cfblk5/1 -> cfblk14/2(cfblk16)
  cfblk7/1 -> cfblk18/1
  cfblk18/1 -> cfblk14/1(cfblk1)
  cfblk9/1 -> cfblk19/1
  cfblk19/1 -> cfblk3/1

== system Sample594/cfblk7/cfblk9/cfblk7 ==
  cfblk1 : Inport
  cfblk7 : Inport  Port=2
  cfblk8 : Inport  Port=3
  cfblk9 : Inport  Port=4
  cfblk10 : Delay  SampleTime=1
  cfblk3 : simulink/Discrete/Transfer Fcn Lead or Lag  PoleZ=0.95  ZeroZ=0.75  ICPrevOutput=0.0  ICPrevInput=0.0  DoSatur=off
      settings: SourceProductBaseCode=SL
  cfblk4 : DotProduct  InputSameDT=on  OutDataTypeStr=Inherit: Inherit via internal rule
  cfblk5 : Sin  TimeSource=Use external signal  SampleTime=0
  cfblk6 : Subsystem
  cfblk2 : Outport
  wires:
  cfblk7/1 -> cfblk6/1(cfblk1)
  cfblk4/1 -> cfblk6/2(cfblk7)
  cfblk3/1 -> cfblk2/1
  cfblk1/1 -> cfblk4/1
  cfblk8/1 -> cfblk3/1, cfblk6/4(cfblk9)
  cfblk6/1(cfblk2) -> cfblk5/1
  cfblk9/1 -> cfblk4/2
  cfblk5/1 -> cfblk10/1
  cfblk10/1 -> cfblk6/3(cfblk8)

== system Sample594/cfblk7/cfblk9/cfblk8 ==
  cfblk1 : Inport
  cfblk10 : Constant  Value=[-985307659.669615]  SampleTime=1
  cfblk11 : Subsystem
  cfblk12 : Subsystem
  cfblk3 : Delay  ShowEnablePort=on  SampleTime=1
      settings: InputPortMap=u0,e6
  cfblk4 : DiscreteTransferFcn  SampleTime=1
  cfblk5 : Product
  cfblk6 : Squeeze
  cfblk7 : Constant  Value=[461093766.238978]  SampleTime=1
  cfblk8 : Constant  Value=[699907887.353104]  SampleTime=1
  cfblk9 : Constant  Value=[92694793.282824]  SampleTime=1
  cfblk2 : Outport
  wires:
  cfblk1/1 -> cfblk3/1
  cfblk6/1 -> cfblk3/2
  cfblk4/1 -> cfblk12/1(cfblk1)
  cfblk7/1 -> cfblk2/1
  cfblk9/1 -> cfblk5/1
  cfblk12/1(cfblk2) -> cfblk11/1(cfblk1)
  cfblk8/1 -> cfblk12/2(cfblk9)
  cfblk5/1 -> cfblk6/1
  cfblk10/1 -> cfblk5/2
  cfblk3/1 -> cfblk4/1
  cfblk12/2(cfblk10) -> cfblk11/2(cfblk12)

== system Sample594/cfblk8/cfblk10/cfblk8 ==
  cfblk1 : Inport
  cfblk12 : Inport  Port=2
  cfblk13 : Inport  Port=3
  cfblk14 : Inport  Port=4
  cfblk10 : Subsystem
  cfblk11 : Subsystem
  cfblk16 : Delay  SampleTime=1
  cfblk3 : simulink/Discrete/Difference  ICPrevInput=0.0  OutMin=[]  OutMax=[]  OutDataTypeStr=Inherit: Inherit via back propagation  OutDataType=fixdt(1, 16)  OutScaling=2^-10  DoSatur=off
  cfblk4 : simulink/Discrete/Transfer Fcn Lead or Lag  PoleZ=0.95  ZeroZ=0.75  ICPrevOutput=0.0  ICPrevInput=0.0  DoSatur=off
      settings: SourceProductBaseCode=SL
  cfblk5 : Sum  Inputs=+-
  cfblk6 : Signum
  cfblk7 : ComplexToMagnitudeAngle
  cfblk8 : Product  Inputs=*
  cfblk9 : Constant  Value=[489290151.517100]  SampleTime=1
  cfblk2 : Outport
  cfblk15 : Outport  Port=2
  wires:
  cfblk4/1 -> cfblk3/1
  cfblk1/1 -> cfblk2/1
  cfblk14/1 -> cfblk4/1
  cfblk11/1(cfblk2) -> cfblk5/1
  cfblk9/1 -> cfblk10/1(cfblk1), cfblk10/3(cfblk11)
  cfblk7/1 -> cfblk5/2
  cfblk13/1 -> cfblk7/1
  cfblk5/1 -> cfblk10/2(cfblk10), cfblk10/4(cfblk12)
  cfblk12/1 -> cfblk15/1
  cfblk7/2 -> cfblk11/2(cfblk6)
  cfblk6/1 -> cfblk8/1
  cfblk3/1 -> cfblk11/3(cfblk7), cfblk10/5(cfblk13)
  cfblk10/1(cfblk2) -> cfblk6/1
  cfblk8/1 -> cfblk16/1
  cfblk16/1 -> cfblk11/1(cfblk1)

== system Sample594/cfblk8/cfblk11/cfblk10 ==
  cfblk1 : Inport
  cfblk11 : Inport  Port=2
  cfblk10 : Constant  Value=[347588637.480266]  SampleTime=1
  cfblk3 : simulink/Discrete/Transfer Fcn Lead or Lag  PoleZ=0.95  ZeroZ=0.75  ICPrevOutput=0.0  ICPrevInput=0.0  DoSatur=off
      settings: SourceProductBaseCode=SL
  cfblk4 : simulink/Discrete/Transfer Fcn Real Zero  ZeroZ=0.75  ICPrevInput=0.0  DoSatur=off
      settings: SourceProductBaseCode=SL
  cfblk5 : pid_lib/PID Controller (2DOF)  Controller=PID  Form=Parallel  TimeDomain=Discrete-time  UseExternalTs=off  SampleTime=1  IntegratorMethod=Forward Euler  FilterMethod=Forward Euler  ControllerParametersSource=internal  P=1  I=1  D=0  UseFilter=on  N=100  b=1  c=1  TunerSelectOption=Transfer Function Based (PID Tuner App)  InitialConditionSource=internal  InitialConditionForIntegrator=0  InitialConditionForFilter=0  DifferentiatorICPrevScaledInput=0  ExternalReset=none  TrackingMode=off  Kt=1  LimitOutput=off  SatLimitsSource=internal  UpperSaturationLimit=inf  LowerSaturationLimit=-inf  LinearizeAsGain=off  AntiWindupMode=none  Kb=1  POutMin=[]  POutMax=[]  IOutMin=[]  IOutMax=[]  DOutMin=[]  DOutMax=[]  NOutMin=[]  NOutMax=[]  bOutMin=[]  bOutMax=[]  cOutMin=[]  cOutMax=[]  SumOutMin=[]  SumOutMax=[]  SaturationOutMin=[]  SaturationOutMax=[]  PParamMin=[]  PParamMax=[]  IParamMin=[]  IParamMax=[]  DParamMin=[]  DParamMax=[]  NParamMin=[]  NParamMax=[]  bParamMin=[]  bParamMax=[]  cParamMin=[]  cParamMax=[]  KbParamMin=[]  KbParamMax=[]  KtParamMin=[]  KtParamMax=[]  KbOutMin=[]  KbOutMax=[]  KtOutMin=[]  KtOutMax=[]  IntegratorOutMin=[]  IntegratorOutMax=[]  FilterOutMin=[]  FilterOutMax=[]  SumI1OutMin=[]  SumI1OutMax=[]  SumI2OutMin=[]  SumI2OutMax=[]  SumI3OutMin=[]  SumI3OutMax=[]  SumI4OutMin=[]  SumI4OutMax=[]  SumDOutMin=[]  SumDOutMax=[]  Sum1OutMin=[]  Sum1OutMax=[]  Sum2OutMin=[]  Sum2OutMax=[]  Sum3OutMin=[]  Sum3OutMax=[]  DifferentiatorOutMin=[]  DifferentiatorOutMax=[]  FilterDiffOutCoefMin=[]  FilterDiffOutCoefMax=[]  ReciprocalOutMin=[]  ReciprocalOutMax=[]  SumDenOutMin=[]  SumDenOutMax=[]  SumNumOutMin=[]  SumNumOutMax=[]  DivideOutMin=[]  DivideOutMax=[]  UdiffTsProdOutMin=[]  UdiffTsProdOutMax=[]  NTsProdOutMin=[]  NTsProdOutMax=[]  UintegralTsProdOutMin=[]  UintegralTsProdOutMax=[]  UngainTsProdOutMin=[]  UngainTsProdOutMax=[]  IntegratorContinuousStateAttributes=''  IntegratorStateMustResolveToSignalObject=off  IntegratorRTWStateStorageClass=Auto  FilterContinuousStateAttributes=''  FilterStateMustResolveToSignalObject=off  FilterRTWStateStorageClass=Auto  ParallelPVariant=InternalParameters  IdealPVariant=Disabled  IVariant=InternalParameters  DVariant=InternalParameters  bVariant=InternalParameters  cVariant=InternalParameters  IntegratorVariant=Discrete  SatVariant=Disabled  AWVariant=Passthrough  PCopyVariant=Disabled  TRVariant=Disabled  FdbkBlocksVariant=Forward  IdealPFdbkVariant=Disabled  SatFdbkVariant=Disabled  DerivativeFilterVariant=ForwardEulerFilter  NVariant=InternalParameters  NCopyVariant=Disabled  FilterICVariant=InternalICsFilter  IntegratorICVariant=InternalICs  ExternalResetVariant=Disabled  TRSumVariant=Passthrough  SumFdbkVariant=Disabled  SumVariant=Sum_PID  TsampFilterVariant=InternalTs  TsampNgainVariant=Passthrough  TsampIntegralVariant=Passthrough  ExternalSaturationOutDataTypeStr=Inherit: Same as second input
      settings: SourceProductBaseCode=SL
  cfblk6 : Delay  ShowEnablePort=on  SampleTime=1
      settings: InputPortMap=u0,e6
  cfblk7 : Math  Operator=log10  SaturateOnIntegerOverflow=on
  cfblk8 : ComplexToMagnitudeAngle
  cfblk9 : Constant  Value=[-665785419.779974]  SampleTime=1
  cfblk2 : Outport
  cfblk12 : Outport  Port=2
  wires:
  cfblk5/1 -> cfblk2/1
  cfblk10/1 -> cfblk12/1
  cfblk9/1 -> cfblk7/1
  cfblk11/1 -> cfblk3/1
  cfblk3/1 -> cfblk4/1
  cfblk1/1 -> cfblk6/1
  cfblk4/1 -> cfblk8/1
  cfblk6/1 -> cfblk5/1
  cfblk8/1 -> cfblk5/2
  cfblk7/1 -> cfblk6/2

== system Sample594/cfblk8/cfblk11/cfblk11 ==
  cfblk1 : Inport
  cfblk13 : Inport  Port=2
  cfblk14 : Inport  Port=3
  cfblk10 : Subsystem
  cfblk11 : Subsystem
  cfblk12 : Subsystem
  cfblk15 : Delay  SampleTime=1
  cfblk16 : Delay  SampleTime=1
  cfblk17 : Delay  SampleTime=1
  cfblk3 : simulink/Discrete/Difference  ICPrevInput=0.0  OutMin=[]  OutMax=[]  OutDataTypeStr=Inherit: Inherit via back propagation  OutDataType=fixdt(1, 16)  OutScaling=2^-10  DoSatur=off
  cfblk4 : pid_lib/PID Controller  Controller=PID  Form=Parallel  TimeDomain=Discrete-time  UseExternalTs=off  SampleTime=1  IntegratorMethod=Forward Euler  FilterMethod=Forward Euler  ControllerParametersSource=internal  P=1  I=1  D=0  UseFilter=on  N=100  TunerSelectOption=Transfer Function Based (PID Tuner App)  InitialConditionSource=internal  InitialConditionForIntegrator=0  InitialConditionForFilter=0  DifferentiatorICPrevScaledInput=0  ExternalReset=none  TrackingMode=off  Kt=1  LimitOutput=off  SatLimitsSource=internal  UpperSaturationLimit=inf  LowerSaturationLimit=-inf  LinearizeAsGain=off  AntiWindupMode=none  Kb=1  POutMin=[]  POutMax=[]  IOutMin=[]  IOutMax=[]  DOutMin=[]  DOutMax=[]  NOutMin=[]  NOutMax=[]  SumOutMin=[]  SumOutMax=[]  SaturationOutMin=[]  SaturationOutMax=[]  PParamMin=[]  PParamMax=[]  IParamMin=[]  IParamMax=[]  DParamMin=[]  DParamMax=[]  NParamMin=[]  NParamMax=[]  KbParamMin=[]  KbParamMax=[]  KtParamMin=[]  KtParamMax=[]  KbOutMin=[]  KbOutMax=[]  KtOutMin=[]  KtOutMax=[]  IntegratorOutMin=[]  IntegratorOutMax=[]  FilterOutMin=[]  FilterOutMax=[]  SumI1OutMin=[]  SumI1OutMax=[]  SumI2OutMin=[]  SumI2OutMax=[]  SumI3OutMin=[]  SumI3OutMax=[]  SumI4OutMin=[]  SumI4OutMax=[]  SumDOutMin=[]  SumDOutMax=[]  DifferentiatorOutMin=[]  DifferentiatorOutMax=[]  FilterDiffOutCoefMin=[]  FilterDiffOutCoefMax=[]  ReciprocalOutMin=[]  ReciprocalOutMax=[]  SumDenOutMin=[]  SumDenOutMax=[]  SumNumOutMin=[]  SumNumOutMax=[]  DivideOutMin=[]  DivideOutMax=[]  UdiffTsProdOutMin=[]  UdiffTsProdOutMax=[]  NTsProdOutMin=[]  NTsProdOutMax=[]  UintegralTsProdOutMin=[]  UintegralTsProdOutMax=[]  UngainTsProdOutMin=[]  UngainTsProdOutMax=[]  IntegratorContinuousStateAttributes=''  IntegratorStateMustResolveToSignalObject=off  IntegratorRTWStateStorageClass=Auto  FilterContinuousStateAttributes=''  FilterStateMustResolveToSignalObject=off  FilterRTWStateStorageClass=Auto  ParallelPVariant=InternalParameters  IdealPVariant=Disabled  IVariant=InternalParameters  DVariant=InternalParameters  IntegratorVariant=Discrete  SatVariant=Disabled  AWVariant=Passthrough  PCopyVariant=Disabled  TRVariant=Disabled  FdbkBlocksVariant=Forward  IdealPFdbkVariant=Disabled  SatFdbkVariant=Disabled  DerivativeFilterVariant=ForwardEulerFilter  NVariant=InternalParameters  NCopyVariant=Disabled  FilterICVariant=InternalICsFilter  IntegratorICVariant=InternalICs  ExternalResetVariant=Disabled  TRSumVariant=Passthrough  SumFdbkVariant=Disabled  SumVariant=Sum_PID  TsampFilterVariant=InternalTs  TsampNgainVariant=Passthrough  TsampIntegralVariant=Passthrough  ExternalSaturationOutDataTypeStr=Inherit: Same as second input
  cfblk5 : ComplexToMagnitudeAngle
  cfblk6 : Sum  Inputs=-+
  cfblk7 : Product
  cfblk8 : Sum  Inputs=+
  cfblk9 : Constant  Value=[607444552.439598]  SampleTime=1
  cfblk2 : Outport
  wires:
  cfblk9/1 -> cfblk7/1
  cfblk7/1 -> cfblk6/1
  cfblk6/1 -> cfblk10/1(cfblk1), cfblk10/4(cfblk9)
  cfblk13/1 -> cfblk3/1
  cfblk12/1(cfblk2) -> cfblk5/1
  cfblk14/1 -> cfblk2/1
  cfblk8/1 -> cfblk6/2, cfblk10/3(cfblk8)
  cfblk11/1(cfblk2) -> cfblk4/1
  cfblk12/2(cfblk16) -> cfblk11/1(cfblk1)
  cfblk12/3(cfblk17) -> cfblk10/2(cfblk7)
  cfblk1/1 -> cfblk12/1(cfblk1)
  cfblk4/1 -> cfblk7/2
  cfblk3/1 -> cfblk8/1
  cfblk5/2 -> cfblk11/3(cfblk8), cfblk10/5(cfblk10)
  cfblk5/1 -> cfblk15/1
  cfblk15/1 -> cfblk12/2(cfblk15)
  cfblk10/1(cfblk2) -> cfblk16/1
  cfblk16/1 -> cfblk11/2(cfblk7)
  cfblk10/2(cfblk11) -> cfblk17/1
  cfblk17/1 -> cfblk11/4(cfblk9)

== system Sample594/cfblk8/cfblk11/cfblk12 ==
  cfblk1 : Inport
  cfblk15 : Inport  Port=2
  cfblk10 : Subsystem
  cfblk11 : Subsystem
  cfblk12 : Subsystem
  cfblk13 : Subsystem
  cfblk14 : Subsystem
  cfblk17 : Delay  SampleTime=1
  cfblk18 : Delay  SampleTime=1
  cfblk3 : simulink/Discrete/Difference  ICPrevInput=0.0  OutMin=[]  OutMax=[]  OutDataTypeStr=Inherit: Inherit via back propagation  OutDataType=fixdt(1, 16)  OutScaling=2^-10  DoSatur=off
  cfblk4 : Product
  cfblk5 : PermuteDimensions
  cfblk6 : Gain  Gain=[-136151742.575265]
  cfblk7 : simulink/Math Operations/MinMax Running Resettable  Function=min  vinit=0.0
  cfblk8 : ComplexToMagnitudeAngle
  cfblk9 : Constant  Value=[-739890555.385763]  SampleTime=1
  cfblk2 : Outport
  cfblk16 : Outport  Port=2
  wires:
  cfblk14/1(cfblk2) -> cfblk2/1, cfblk7/2
  cfblk12/1(cfblk2) -> cfblk14/1(cfblk1)
  cfblk15/1 -> cfblk6/1
  cfblk10/1(cfblk2) -> cfblk12/1(cfblk1)
  cfblk7/1 -> cfblk3/1
  cfblk8/1 -> cfblk7/1
  cfblk11/1(cfblk2) -> cfblk5/1
  cfblk3/1 -> cfblk11/2(cfblk14)
  cfblk8/2 -> cfblk14/2(cfblk11), cfblk12/2(cfblk10)
  cfblk6/1 -> cfblk4/1
  cfblk11/2(cfblk15) -> cfblk4/2
  cfblk13/1(cfblk2) -> cfblk8/1, cfblk16/1, cfblk10/1(cfblk1)
  cfblk1/1 -> cfblk13/2(cfblk10)
  cfblk9/1 -> cfblk13/3(cfblk11)
  cfblk5/1 -> cfblk17/1
  cfblk17/1 -> cfblk13/1(cfblk1)
  cfblk4/1 -> cfblk18/1
  cfblk18/1 -> cfblk11/1(cfblk1)

== system Sample594/cfblk8/cfblk11/cfblk9 ==
  cfblk1 : Inport
  cfblk6 : Inport  Port=2
  cfblk3 : Subsystem
  cfblk4 : Subsystem
  cfblk5 : Subsystem
  cfblk9 : Delay  SampleTime=1
  cfblk2 : Outport
  cfblk7 : Outport  Port=2
  cfblk8 : Outport  Port=3
  wires:
  cfblk6/1 -> cfblk5/1(cfblk1)
  cfblk4/1(cfblk2) -> cfblk3/1(cfblk1)
  cfblk4/2(cfblk12) -> cfblk7/1
  cfblk5/1(cfblk2) -> cfblk2/1
  cfblk1/1 -> cfblk8/1, cfblk5/3(cfblk15)
  cfblk5/2(cfblk16) -> cfblk3/2(cfblk8), cfblk4/1(cfblk1), cfblk4/2(cfblk11)
  cfblk3/1(cfblk2) -> cfblk9/1
  cfblk9/1 -> cfblk5/2(cfblk14)

== system Sample594/cfblk8/cfblk12/cfblk10 ==
  cfblk1 : Inport
  cfblk10 : Subsystem
  cfblk11 : Subsystem
  cfblk12 : If  IfExpression=u1 >= 0  SampleTime=1
  cfblk13 : Subsystem  TreatAsAtomicUnit=on
  cfblk14 : Subsystem  TreatAsAtomicUnit=on
  cfblk{15..20} (6 alike) : Delay  SampleTime=1
  cfblk3 : DiscreteIntegrator  ICPrevOutput=DiscIntNeverNeededParam  ICPrevScaledInput=DiscIntNeverNeededParam
  cfblk4 : simulink/Math Operations/MinMax Running Resettable  Function=min  vinit=0.0
  cfblk5 : Product  Inputs=**
  cfblk6 : Product
  cfblk7 : Subsystem
  cfblk8 : Subsystem
  cfblk9 : Subsystem
  cfblk2 : Outport
  wires:
  cfblk4/1 -> cfblk10/1(cfblk1)
  cfblk8/1(cfblk2) -> cfblk2/1
  cfblk7/1(cfblk2) -> cfblk9/2(cfblk12), cfblk9/4(cfblk14), cfblk17/1
  cfblk11/2(cfblk8) -> cfblk8/1(cfblk1)
  cfblk13/1(cfblk2) -> cfblk5/1
  cfblk13/2(cfblk7) -> cfblk6/1
  cfblk10/1(cfblk2) -> cfblk14/1(cfblk1), cfblk7/3(cfblk11)
  cfblk14/3(cfblk11) -> cfblk3/1, cfblk11/2(cfblk7)
  cfblk1/1 -> cfblk4/2, cfblk14/2(cfblk9)
  cfblk3/1 -> cfblk5/2
  cfblk9/1(cfblk2) -> cfblk6/2
  cfblk5/1 -> cfblk11/1(cfblk1), cfblk9/3(cfblk13), cfblk18/1
  cfblk8/2(cfblk7) -> cfblk7/1(cfblk1)
  cfblk13/3(cfblk8) -> cfblk7/2(cfblk10)
  cfblk12/1 -> cfblk13/Action
  cfblk12/2 -> cfblk14/Action
  cfblk11/1(cfblk2) -> cfblk15/1
  cfblk15/1 -> cfblk4/1
  cfblk6/1 -> cfblk16/1
  cfblk16/1 -> cfblk9/1(cfblk1)
  cfblk17/1 -> cfblk13/2(cfblk6)
  cfblk18/1 -> cfblk13/1(cfblk1)
  cfblk14/1(cfblk2) -> cfblk19/1
  cfblk19/1 -> cfblk12/1
  cfblk14/2(cfblk10) -> cfblk20/1
  cfblk20/1 -> cfblk10/2(cfblk7)

== system Sample594/cfblk8/cfblk12/cfblk11 ==
  cfblk1 : Inport
  cfblk10 : Delay  SampleTime=1
  cfblk3 : Sqrt  SaturateOnIntegerOverflow=on
  cfblk4 : Constant  Value=[609084039.271213]  SampleTime=1
  cfblk5 : Subsystem
  cfblk6 : Subsystem
  cfblk7 : Subsystem
  cfblk8 : Subsystem
  cfblk9 : Delay  SampleTime=1
  cfblk2 : Outport
  wires:
  cfblk5/1(cfblk2) -> cfblk3/1
  cfblk4/1 -> cfblk7/1(cfblk1)
  cfblk7/1(cfblk2) -> cfblk8/1(cfblk1)
  cfblk1/1 -> cfblk5/1(cfblk1)
  cfblk6/1(cfblk2) -> cfblk7/2(cfblk7)
  cfblk5/2(cfblk8) -> cfblk2/1
  cfblk5/3(cfblk9) -> cfblk6/2(cfblk10)
  cfblk8/1(cfblk2) -> cfblk9/1
  cfblk9/1 -> cfblk5/2(cfblk7)
  cfblk7/2(cfblk8) -> cfblk10/1
  cfblk10/1 -> cfblk6/1(cfblk1)

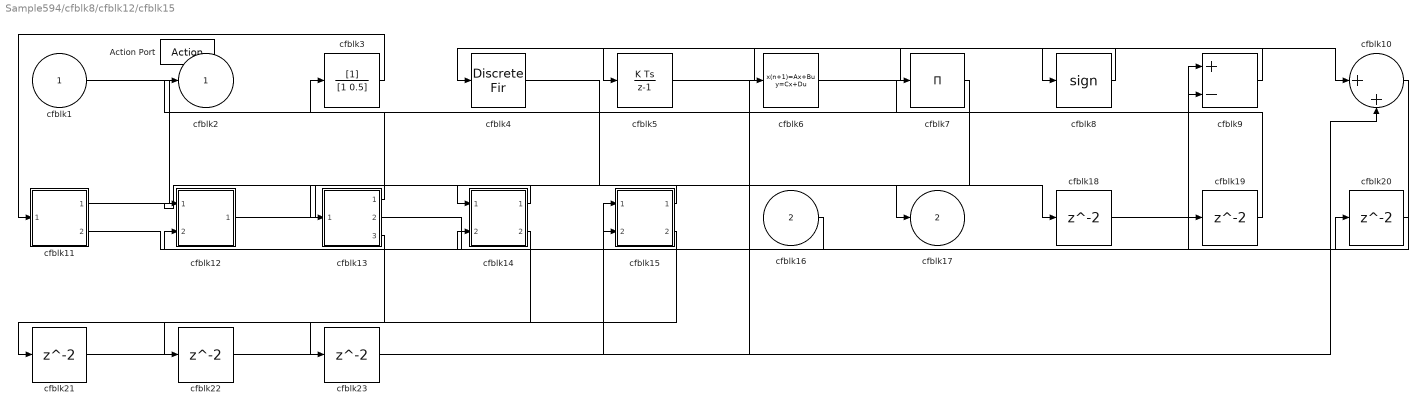
== system Sample594/cfblk8/cfblk12/cfblk15 ==
  cfblk1 : Inport
  cfblk16 : Inport  Port=2
  Action Port : ActionPort  ActionPortLabel=if(u1 >= 0)
  cfblk10 : Sum  Inputs=|++
  cfblk11 : Subsystem
  cfblk12 : Subsystem
  cfblk13 : Subsystem
  cfblk14 : Subsystem
  cfblk15 : Subsystem
  cfblk{18..23} (6 alike) : Delay
  cfblk3 : DiscreteFilter
  cfblk4 : DiscreteFir
  cfblk5 : DiscreteIntegrator  SampleTime=-1  ICPrevOutput=DiscIntNeverNeededParam  ICPrevScaledInput=DiscIntNeverNeededParam
  cfblk6 : DiscreteStateSpace  SampleTime=-1
  cfblk7 : Product  Inputs=*
  cfblk8 : Signum
  cfblk9 : Sum  Inputs=+-
  cfblk2 : Outport
  cfblk17 : Outport  Port=2
  wires:
  cfblk11/1(cfblk2) -> cfblk9/1
  cfblk9/1 -> cfblk5/1
  cfblk6/1 -> cfblk10/1
  cfblk15/1(cfblk2) -> cfblk12/1(cfblk1)
  cfblk8/1 -> cfblk4/1
  cfblk10/1 -> cfblk15/1(cfblk1)
  cfblk3/1 -> cfblk11/1(cfblk1)
  cfblk16/1 -> cfblk12/2(cfblk12)
  cfblk7/1 -> cfblk17/1
  cfblk1/1 -> cfblk7/1
  cfblk5/1 -> cfblk8/1
  cfblk13/1(cfblk2) -> cfblk2/1
  cfblk12/1(cfblk2) -> cfblk14/1(cfblk1)
  cfblk14/1(cfblk2) -> cfblk13/1(cfblk1)
  cfblk4/1 -> cfblk18/1
  cfblk18/1 -> cfblk9/2
  cfblk11/2(cfblk14) -> cfblk19/1
  cfblk19/1 -> cfblk3/1
  cfblk13/2(cfblk6) -> cfblk20/1
  cfblk20/1 -> cfblk14/2(cfblk9)
  cfblk13/3(cfblk7) -> cfblk21/1
  cfblk21/1 -> cfblk10/2
  cfblk14/2(cfblk10) -> cfblk22/1
  cfblk22/1 -> cfblk15/2(cfblk12)
  cfblk15/2(cfblk13) -> cfblk23/1
  cfblk23/1 -> cfblk6/1

== system Sample594/cfblk8/cfblk12/cfblk16 ==
  cfblk1 : Inport
  cfblk16 : Inport  Port=2
  cfblk17 : Inport  Port=3
  Action Port : ActionPort  ActionPortLabel=else
  cfblk10 : DotProduct  InputSameDT=on  OutDataTypeStr=Inherit: Inherit via internal rule
  cfblk11 : Constant  Value=[681045932.606803]  SampleTime=1
  cfblk12 : Constant  Value=[615265013.536704]  SampleTime=1
  cfblk13 : Constant  Value=[149751800.512534]  SampleTime=1
  cfblk14 : Subsystem
  cfblk15 : If  IfExpression=u1 >= 0  SampleTime=1
  cfblk18 : Subsystem  TreatAsAtomicUnit=on
  cfblk19 : Subsystem  TreatAsAtomicUnit=on
  cfblk20 : Delay
  cfblk21 : Delay
  cfblk3 : Squeeze
  cfblk4 : Signum
  cfblk5 : simulink/Math Operations/Slider Gain  gain=1  low=0  high=2
  cfblk6 : Product  Inputs=**
  cfblk7 : simulink/Math Operations/Slider Gain  gain=1  low=0  high=2
  cfblk8 : simulink/Math Operations/MinMax Running Resettable  Function=min  vinit=0.0
  cfblk9 : Squeeze
  cfblk2 : Outport
  wires:
  cfblk1/1 -> cfblk14/1(cfblk1)
  cfblk6/1 -> cfblk5/1
  cfblk16/1 -> cfblk6/1
  cfblk3/1 -> cfblk6/2
  cfblk11/1 -> cfblk14/2(cfblk14)
  cfblk17/1 -> cfblk18/2(cfblk7)
  cfblk19/1(cfblk2) -> cfblk8/1
  cfblk10/1 -> cfblk2/1
  cfblk4/1 -> cfblk9/1
  cfblk12/1 -> cfblk18/3(cfblk8)
  cfblk13/1 -> cfblk10/1
  cfblk5/1 -> cfblk4/1
  cfblk18/1(cfblk2) -> cfblk3/1
  cfblk18/2(cfblk9) -> cfblk10/2
  cfblk7/1 -> cfblk8/2
  cfblk14/1(cfblk2) -> cfblk15/1
  cfblk14/2(cfblk15) -> cfblk7/1
  cfblk15/1 -> cfblk18/Action
  cfblk15/2 -> cfblk19/Action
  cfblk9/1 -> cfblk20/1
  cfblk20/1 -> cfblk19/1(cfblk1)
  cfblk8/1 -> cfblk21/1
  cfblk21/1 -> cfblk18/1(cfblk1)

== system Sample594/cfblk8/cfblk12/cfblk9 ==
  cfblk1 : Inport
  cfblk10 : Subsystem
  cfblk13 : Delay  SampleTime=1
  cfblk3 : UnitDelay  HasFrameUpgradeWarning=on
  cfblk4 : DiscreteStateSpace
  cfblk5 : UnitDelay  HasFrameUpgradeWarning=on
  cfblk6 : Gain  Gain=[64531892.813032]
  cfblk7 : Rounding
  cfblk8 : Subsystem
  cfblk9 : Subsystem
  cfblk2 : Outport
  cfblk11 : Outport  Port=2
  cfblk12 : Outport  Port=3
  wires:
  cfblk8/1(cfblk2) -> cfblk7/1
  cfblk1/1 -> cfblk6/1, cfblk10/2(cfblk13)
  cfblk10/1(cfblk2) -> cfblk4/1
  cfblk4/1 -> cfblk2/1
  cfblk3/1 -> cfblk5/1
  cfblk7/1 -> cfblk3/1
  cfblk9/1(cfblk2) -> cfblk11/1
  cfblk9/2(cfblk9) -> cfblk10/1(cfblk1)
  cfblk5/1 -> cfblk12/1
  cfblk6/1 -> cfblk9/1(cfblk1)
  cfblk10/2(cfblk14) -> cfblk8/1(cfblk1)
  cfblk10/3(cfblk15) -> cfblk13/1
  cfblk13/1 -> cfblk9/2(cfblk8)

== system Sample594/cfblk8/cfblk13/cfblk5 ==
  cfblk1 : Inport
  cfblk8 : Inport  Port=2
  cfblk10 : Delay  SampleTime=1
  cfblk3 : simulink/Discrete/Transfer Fcn Lead or Lag  PoleZ=0.95  ZeroZ=0.75  ICPrevOutput=0.0  ICPrevInput=0.0  DoSatur=off
      settings: SourceProductBaseCode=SL
  cfblk4 : DiscreteFilter  SampleTime=1
  cfblk5 : Rounding
  cfblk6 : Reshape
  cfblk7 : Subsystem
  cfblk2 : Outport
  cfblk9 : Outport  Port=2
  wires:
  cfblk8/1 -> cfblk6/1
  cfblk1/1 -> cfblk7/1(cfblk1)
  cfblk4/1 -> cfblk2/1
  cfblk6/1 -> cfblk3/1, cfblk9/1
  cfblk3/1 -> cfblk7/3(cfblk8)
  cfblk7/1(cfblk2) -> cfblk5/1
  cfblk7/2(cfblk9) -> cfblk4/1
  cfblk5/1 -> cfblk10/1
  cfblk10/1 -> cfblk7/2(cfblk7)

== system Sample594/cfblk8/cfblk9/cfblk10 ==
  cfblk1 : Inport
  cfblk{9..14} (6 alike) : Delay  SampleTime=1
  cfblk3 : simulink/Discrete/Transfer Fcn Real Zero  ZeroZ=0.75  ICPrevInput=0.0  DoSatur=off
      settings: SourceProductBaseCode=SL
  cfblk4 : Product
  cfblk5 : Subsystem
  cfblk6 : Subsystem
  cfblk7 : Subsystem
  cfblk8 : Subsystem
  cfblk2 : Outport
  wires:
  cfblk6/1(cfblk2) -> cfblk10/1, cfblk11/1, cfblk12/1
  cfblk4/1 -> cfblk6/1(cfblk1)
  cfblk5/1(cfblk2) -> cfblk2/1
  cfblk8/1(cfblk2) -> cfblk7/1(cfblk1), cfblk4/1
  cfblk7/1(cfblk2) -> cfblk5/1(cfblk1)
  cfblk5/2(cfblk12) -> cfblk6/2(cfblk7), cfblk9/1, cfblk13/1
  cfblk1/1 -> cfblk8/3(cfblk10)
  cfblk7/2(cfblk8) -> cfblk3/1, cfblk4/2
  cfblk9/1 -> cfblk7/2(cfblk6)
  cfblk10/1 -> cfblk8/1(cfblk1)
  cfblk11/1 -> cfblk8/4(cfblk11)
  cfblk12/1 -> cfblk8/5(cfblk12)
  cfblk13/1 -> cfblk7/3(cfblk7)
  cfblk3/1 -> cfblk14/1
  cfblk14/1 -> cfblk8/2(cfblk9)

== system Sample594/cfblk8/cfblk9/cfblk6 ==
  cfblk1 : Inport
  cfblk8 : Inport  Port=2
  cfblk9 : Inport  Port=3
  cfblk10 : Inport  Port=4
  cfblk11 : Inport  Port=5
  cfblk12 : Delay  SampleTime=1
  cfblk13 : Delay  SampleTime=1
  cfblk3 : Product
  cfblk4 : Squeeze
  cfblk5 : Subsystem
  cfblk6 : Subsystem
  cfblk7 : Subsystem
  cfblk2 : Outport
  wires:
  cfblk10/1 -> cfblk6/1(cfblk1), cfblk6/5(cfblk14)
  cfblk4/1 -> cfblk7/1(cfblk1), cfblk6/6(cfblk15)
  cfblk3/1 -> cfblk6/2(cfblk11)
  cfblk8/1 -> cfblk3/1
  cfblk6/2(cfblk16) -> cfblk2/1
  cfblk7/1(cfblk2) -> cfblk5/2(cfblk11)
  cfblk9/1 -> cfblk3/2
  cfblk1/1 -> cfblk4/1
  cfblk5/1(cfblk2) -> cfblk6/3(cfblk12)
  cfblk11/1 -> cfblk6/4(cfblk13), cfblk7/2(cfblk8)
  cfblk6/1(cfblk2) -> cfblk12/1
  cfblk12/1 -> cfblk5/1(cfblk1)
  cfblk6/3(cfblk17) -> cfblk13/1
  cfblk13/1 -> cfblk5/3(cfblk12)

== system Sample594/cfblk8/cfblk9/cfblk7 ==
  cfblk1 : Inport
  cfblk9 : Inport  Port=2
  cfblk10 : Inport  Port=3
  cfblk11 : Delay  SampleTime=1
  cfblk3 : simulink/Discrete/Tapped Delay  vinit=0.0  samptime=-1  NumDelays=1  DelayOrder=Oldest  includeCurrent=off
  cfblk4 : simulink/Discrete/Transfer Fcn Real Zero  ZeroZ=0.75  ICPrevInput=0.0  DoSatur=off
      settings: SourceProductBaseCode=SL
  cfblk5 : Abs
  cfblk6 : DotProduct  InputSameDT=on  OutDataTypeStr=Inherit: Inherit via internal rule
  cfblk7 : Subsystem
  cfblk8 : Subsystem
  cfblk2 : Outport
  wires:
  cfblk9/1 -> cfblk5/1
  cfblk1/1 -> cfblk6/2, cfblk7/4(cfblk8)
  cfblk4/1 -> cfblk8/1(cfblk1)
  cfblk8/1(cfblk2) -> cfblk2/1
  cfblk10/1 -> cfblk7/1(cfblk1)
  cfblk5/1 -> cfblk4/1
  cfblk7/1(cfblk2) -> cfblk3/1
  cfblk6/1 -> cfblk7/2(cfblk6), cfblk7/3(cfblk7)
  cfblk3/1 -> cfblk11/1
  cfblk11/1 -> cfblk6/1
